simulink model "comunication"  (R2024b)
settings: Solver=VariableStepAuto  StartTime=0.0  StopTime=inf  FixedStep=0.02  RelTol=1e-3
libraries: opcualib x2
settings Model: Creator=ribei  LastModifiedBy=ribei

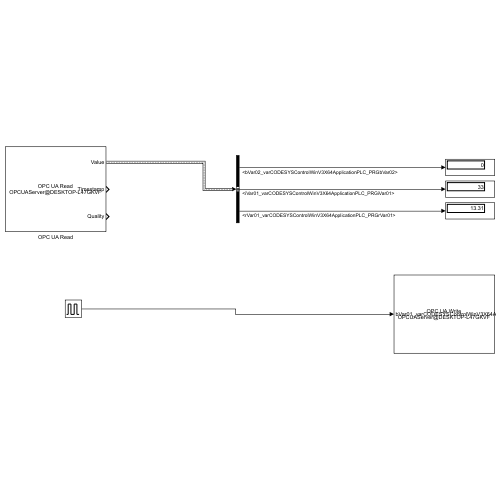
[thumbnail: Simulink's stored preview of the top-level diagram]
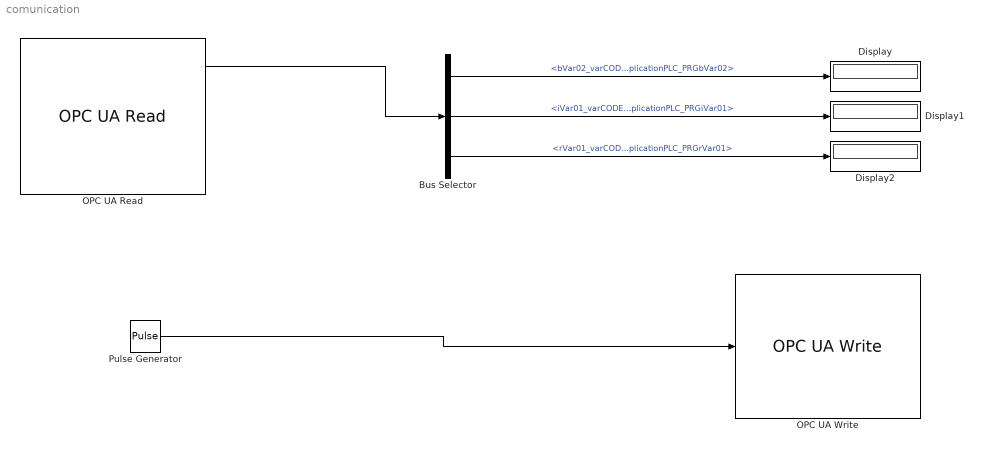
== system comunication ==
  Bus Selector : BusSelector  OutputSignals=bVar02_varCODESYSControlWinV3X64ApplicationPLC_PRGbVar02,iVar01_varCODESYSControlWinV3X64ApplicationPLC_PRGiVar01,rVar01_varCODESYSControlWinV3X64ApplicationPLC_PRGrVar01
  Display : Display
  Display1 : Display
  Display2 : Display
  OPC UA Read : opcualib/OPC UA Read  SelectedServer=OPCUAServer@DESKTOP-L47GKVF  ServerList=OPCUAServer@DESKTOP-L47GKVF  NodeList={ '1', 'bVar02', '4', '|var|CODESYS Control Win V3 x64.Application.PLC_PRG.bVar02', '0'; '2', 'iVar01', '4', '|var|CODESYS Control Win V3 x64.Application.PLC_PRG.iVar01', '0'; '3', 'rVar01', '4', '|var|CODESYS Control Win V3 x64.Application.PLC_PRG.rVar01', '0' }  ShowQualityPort=on  ShowTimestampPort=on  ShowTimestampPortAs=Seconds since start  SampleTime=-1
  OPC UA Write : opcualib/OPC UA Write  SelectedServer=OPCUAServer@DESKTOP-L47GKVF  ServerList=OPCUAServer@DESKTOP-L47GKVF  SampleTime=-1  NodeList={ '1', 'bVar01', '4', '|var|CODESYS Control Win V3 x64.Application.PLC_PRG.bVar01', '0' }
  Pulse Generator : DiscretePulseGenerator  PulseType=Time based  PulseWidth=50
  wires:
  OPC UA Read/1 -> Bus Selector/1
  Bus Selector/1 -> Display/1  "<bVar02_varCODESYSControlWinV3X64ApplicationPLC_PRGbVar02>"
  Bus Selector/2 -> Display1/1  "<iVar01_varCODESYSControlWinV3X64ApplicationPLC_PRGiVar01>"
  Bus Selector/3 -> Display2/1  "<rVar01_varCODESYSControlWinV3X64ApplicationPLC_PRGrVar01>"
  Pulse Generator/1 -> OPC UA Write/1
